simulink model "AircraftModel"  (R2022b)
settings: Solver=VariableStepAuto  StartTime=0.0  StopTime=20  MaxStep=0.1  EnableMultiTasking=on
PreLoadFcn:
  | % Parameters
  | Za = -0.2742;
  | Ma = -0.7402;
  | Mq = -0.3710;
  | Zde = -0.0147;
  | Mde = -0.5754;
libraries: SignalEditorBlockLib x1
settings Model: Creator=nicholas  LastModifiedBy=bensweet
settings SolverCC: AlgebraicLoopSolver=TrustRegion  MaxZcPerStep=1
settings DataIOCC: LimitDataPoints=on  ReturnWorkspaceOutputs=off  SignalLoggingName=sigsOut
settings OptimizationCC: ExpressionDepthLimit=2147483647  InitFltsAndDblsToZero=on  LifeSpan=inf
settings DebuggingCC: UnconnectedInputMsg=warning  UnconnectedOutputMsg=warning  UnconnectedLineMsg=warning  PregeneratedLibrarySubsystemCodeDiagnostic=none  SFMachineParentedDataDiag=warning
settings HardwareCC: ProdBitPerPointer=32  ProdBitPerSizeT=32  ProdBitPerPtrDiffT=32  ProdLargestAtomicFloat=None  ProdIntDivRoundTo=Undefined  ProdEndianess=Unspecified  ProdWordSize=32  ProdHWDeviceType=32-bit Generic  TargetUnknown=on
settings ModelReferenceCC: EnableRefExpFcnMdlSchedulingChecks=on  PropagateSignalLabelsOutOfModel=off
settings SFSimCC: SimUseLocalCustomCode=off
settings RTWCC: RTWUseLocalCustomCode=off  DLArmComputeVersion=19.05
settings CodeAppCC: StateflowObjectComments=on
settings GRTTargetCC: TargetFcnLib=ansi_tfl_tmw.mat  TargetLangStandard=C89/C90 (ANSI)  CombineOutputUpdateFcns=off  GRTInterface=on
settings ConfigComp: CovMetricSettings=dw  CovSaveCumulativeToWorkspaceVar=on  CovSaveSingleToWorkspaceVar=on  CovExternalEMLEnable=off  CovSFcnEnable=off

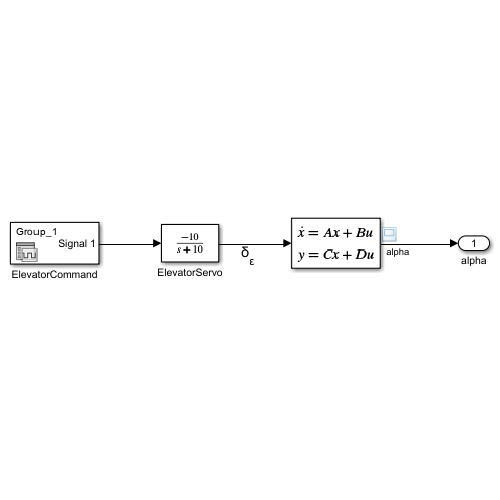
[thumbnail: Simulink's stored preview of the top-level diagram]
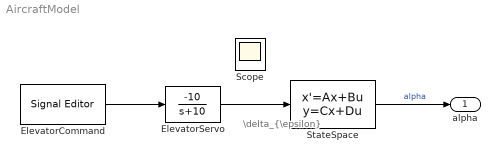
== system AircraftModel ==
  note: \delta_{\epsilon}
  ElevatorCommand : SignalEditorBlockLib/Signal Editor  FileName=AircraftModel_ElevatorCommand_dataset.mat  ActiveScenario=Group_1  ActiveSignal=Signal 1  IsBus=off  OutputBusObjectStr=Bus: BusObject  SampleTime=0  OutputAfterFinalValue=Extrapolation  Unit=inherit  PreserveSignalName=on
  ElevatorServo : TransferFcn  Numerator=[-10]  Denominator=[1 10]
  StateSpace : StateSpace  A=[Za 1;Ma Mq]  B=[Zde;Mde]  C=[1 0]  D=0  InitialCondition=0
  alpha : Outport  VectorParamsAs1DForOutWhenUnconnected=off
  Scope : Scope
  wires:
  ElevatorCommand/1 -> ElevatorServo/1
  ElevatorServo/1 -> StateSpace/1
  StateSpace/1 -> alpha/1  "alpha"
